simulink model "banco_pid"  (Simulink 5.0)
settings: Solver=ode45  StartTime=0.0  StopTime=10.0  RelTol=1e-3
libraries: simulink_extras x4
settings Model: LastModifiedBy=-

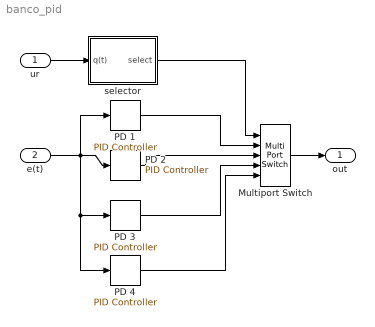
== system banco_pid ==
  ur : Inport
  e(t) : Inport  Port=2
  Multiport Switch : MultiPortSwitch  SaturateOnIntegerOverflow=on
  PD 1 : simulink_extras/Additional Linear/PID Controller  P=111  I=0  D=158.73
  PD 2 : simulink_extras/Additional Linear/PID Controller  P=12.34  I=0  D=18.22
  PD 3 : simulink_extras/Additional Linear/PID Controller  P=4.44  I=0  D=6.76
  PD 4 : simulink_extras/Additional Linear/PID Controller  P=2.5  I=0  D=3.9
  selector : Subsystem
  out : Outport
  wires:
  e(t)/1 -> PD 2/1, PD 1/1, PD 3/1, PD 4/1
  PD 1/1 -> Multiport Switch/2
  PD 2/1 -> Multiport Switch/3
  PD 3/1 -> Multiport Switch/4
  Multiport Switch/1 -> out/1
  ur/1 -> selector/1(q(t))
  selector/1(select) -> Multiport Switch/1
  PD 4/1 -> Multiport Switch/5

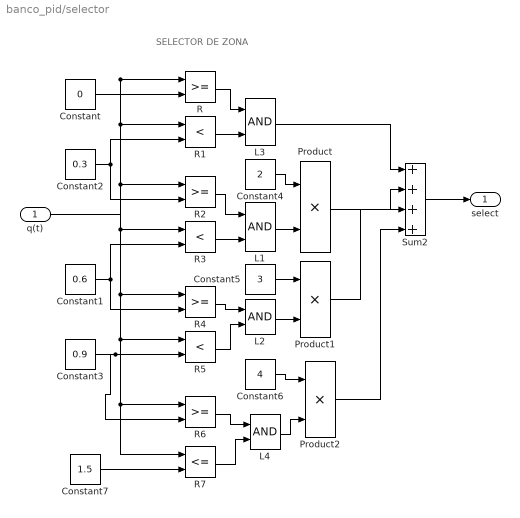
== system banco_pid/selector ==
  note: SELECTOR DE ZONA
  q(t) : Inport
  Constant : Constant  Value=0
  Constant1 : Constant  Value=0.6
  Constant2 : Constant  Value=0.3
  Constant3 : Constant  Value=0.9
  Constant4 : Constant  Value=2
  Constant5 : Constant  Value=3
  Constant6 : Constant  Value=4
  Constant7 : Constant  Value=1.5
  L{1..4} (4 alike) : Logic  AllPortsSameDT=off
  Product : Product  SaturateOnIntegerOverflow=on
  Product1 : Product  SaturateOnIntegerOverflow=on
  Product2 : Product  SaturateOnIntegerOverflow=on
  R{,2,4,6} (4 alike) : RelationalOperator
  R1 : RelationalOperator  Operator=<
  R3 : RelationalOperator  Operator=<
  R5 : RelationalOperator  Operator=<
  R7 : RelationalOperator  Operator=<=
  Sum2 : Sum  Inputs=|++++  SaturateOnIntegerOverflow=on
  select : Outport
  wires:
  Constant/1 -> R/2
  q(t)/1 -> R/1, R1/1, R2/1, R3/1, R4/1, R5/1, R6/1, R7/1
  R/1 -> L3/1
  Constant2/1 -> R1/2, R2/2
  R1/1 -> L3/2
  Constant1/1 -> R3/2, R4/2
  R2/1 -> L1/1
  R3/1 -> L1/2
  Constant3/1 -> R5/2, R6/2
  R5/1 -> L2/2
  Constant4/1 -> Product/1
  L1/1 -> Product/2
  Constant5/1 -> Product1/1
  L2/1 -> Product1/2
  L3/1 -> Sum2/1
  Product/1 -> Sum2/2
  Product1/1 -> Sum2/3
  Sum2/1 -> select/1
  R4/1 -> L2/1
  Constant7/1 -> R7/2
  R7/1 -> L4/2
  L4/1 -> Product2/2
  Product2/1 -> Sum2/4
  R6/1 -> L4/1
  Constant6/1 -> Product2/1
